simulink model "Power_Law_Adaptation"  (R2019a)
settings: Solver=VariableStepAuto  StartTime=0.0  StopTime=testtime  RelTol=1e-3
InitFcn:
  | Power_Law_Test_Parameters
StopFcn:
  | Verify_Power_Law_Adaptation
values from neighbouring files (symbols this model uses):
  alpha1 = 1.5e-6*100e3    (= 0.15)    [PowerLaw.m]    (also in Power_Law_Test_Parameters.m)
  alpha2 = 1e-2*100e3    (= 1000)    [PowerLaw.m]    (also in Power_Law_Test_Parameters.m)
  Fs = 48e3    (= 48000)    [Power_Law_Test_Parameters.m]
undefined symbols (not defined in the file or in its folder): dfilt
libraries: dsparch4 x2, dspsrcs4 x2
settings Model: Creator=mblun  LastModifiedBy=mblun

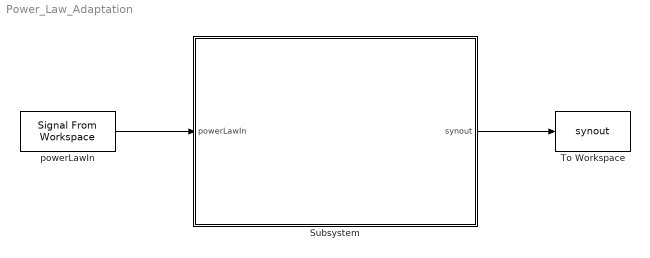
== system Power_Law_Adaptation ==
  Subsystem : Subsystem
  To Workspace : ToWorkspace  VariableName=synout  SampleTime=-1
      settings: Save2DSignal=2-D array (concatenate along first dimension)
  "powerLawIn " : dspsrcs4/Signal From Workspace  X=RxSignal  Ts=1/Fs  nsamps=1  OutputAfterFinalValue=Setting to zero  ignoreOrWarnInputAndFrameLengths=off  OutputFrames=off
  wires:
  "powerLawIn "/1 -> Subsystem/1(powerLawIn)
  Subsystem/1(synout) -> To Workspace/1

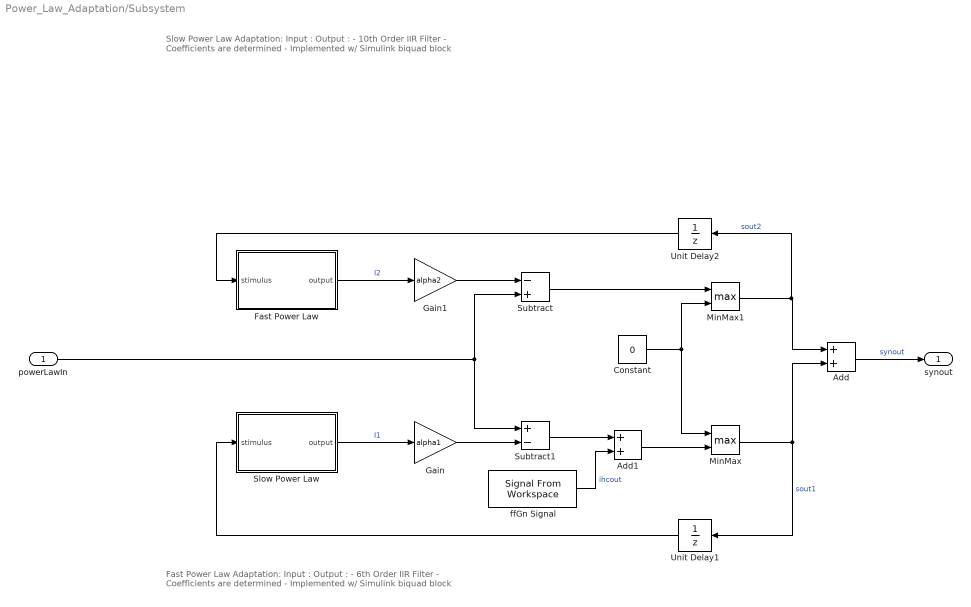
== system Power_Law_Adaptation/Subsystem ==
  note: Fast Power Law Adaptation:
      |
      | Input :
      |
      | Output :
      |
      | - 6th Order IIR Filter
      |
      | - Coefficients are determined
      |
      | - Implemented w/ Simulink biquad block
  note: Slow Power Law Adaptation:
      |
      | Input :
      |
      | Output :
      |
      | - 10th Order IIR Filter
      |
      | - Coefficients are determined
      |
      | - Implemented w/ Simulink biquad block
  powerLawIn : Inport
  Add : Sum
  Add1 : Sum
  Constant : Constant  Value=0  SampleTime=-1
  Fast Power Law : Subsystem
  Gain : Gain  Gain=alpha1
  Gain1 : Gain  Gain=alpha2
  MinMax : MinMax  Function=max  Inputs=2
  MinMax1 : MinMax  Function=max  Inputs=2
  Slow Power Law : Subsystem
  Subtract : Sum  Inputs=-+
  Subtract1 : Sum  Inputs=+-
  Unit Delay1 : UnitDelay  SampleTime=-1  HasFrameUpgradeWarning=on
  Unit Delay2 : UnitDelay  SampleTime=-1  HasFrameUpgradeWarning=on
  ffGn Signal : dspsrcs4/Signal From Workspace  X=randNums  Ts=1/Fs  nsamps=1  OutputAfterFinalValue=Setting to zero  ignoreOrWarnInputAndFrameLengths=off  OutputFrames=off
  synout : Outport
  wires:
  Gain/1 -> Subtract1/2
  Subtract/1 -> MinMax1/1
  MinMax1/1 -> Unit Delay2/1, Add/1  "sout2"
  Add/1 -> synout/1  "synout"
  powerLawIn/1 -> Subtract/2, Subtract1/1
  Fast Power Law/1(output) -> Gain1/1  "I2"
  Unit Delay2/1 -> Fast Power Law/1(stimulus)
  Slow Power Law/1(output) -> Gain/1  "I1"
  Subtract1/1 -> Add1/1
  Constant/1 -> MinMax/1, MinMax1/2
  MinMax/1 -> Unit Delay1/1, Add/2  "sout1"
  Unit Delay1/1 -> Slow Power Law/1(stimulus)
  Gain1/1 -> Subtract/1
  Add1/1 -> MinMax/2
  ffGn Signal/1 -> Add1/2  "ihcout"

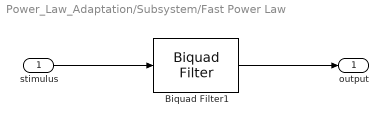
== system Power_Law_Adaptation/Subsystem/Fast Power Law ==
  stimulus : Inport
  Biquad Filter1 : dsparch4/Biquad Filter  FilterSource=Dialog parameters  CoeffSource=Specify via dialog  FilterObject=dfilt.df2tsos([1 0.3 0.4],[1 0.1 0.2])  IIRFiltStruct=Direct form I  BiQuadCoeffs=fast_coeffs  ScaleValues=1  IC=0  ICnum=0  ICden=0  a0Flag=Warning  optimizeScaleValues=on  ScaleValueMode=Specify via input port (g)  roundingMode=Floor  overflowMode=on  scaleValueFracLength=14  denProdOutputFracLength=30  denAccumFracLength=30  secondMemoryFracLength=15
      settings: SourceProductName=DSP System Toolbox
  output : Outport
  wires:
  stimulus/1 -> Biquad Filter1/1
  Biquad Filter1/1 -> output/1

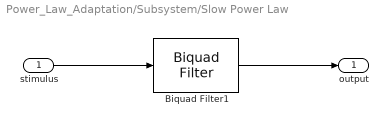
== system Power_Law_Adaptation/Subsystem/Slow Power Law ==
  stimulus : Inport
  Biquad Filter1 : dsparch4/Biquad Filter  FilterSource=Dialog parameters  CoeffSource=Specify via dialog  FilterObject=dfilt.df2tsos([1 0.3 0.4],[1 0.1 0.2])  IIRFiltStruct=Direct form I  BiQuadCoeffs=slow_coeffs  ScaleValues=1  IC=0  ICnum=0  ICden=0  a0Flag=Warning  optimizeScaleValues=on  ScaleValueMode=Specify via input port (g)  roundingMode=Floor  overflowMode=on  scaleValueFracLength=14  denProdOutputFracLength=30  denAccumFracLength=30  secondMemoryFracLength=15
      settings: SourceProductName=DSP System Toolbox
  output : Outport
  wires:
  stimulus/1 -> Biquad Filter1/1
  Biquad Filter1/1 -> output/1
